simulink model "tut1_screwabouts"  (R2023b)
settings: Solver=VariableStepAuto  StartTime=0.0  StopTime=60  RelTol=1e-3
model workspace (MAT data in the model file):
  c = 1
  m = 1000
libraries: slpidlib x1, simulink x1
settings Model: Creator=Matthew  LastModifiedBy=Matthew

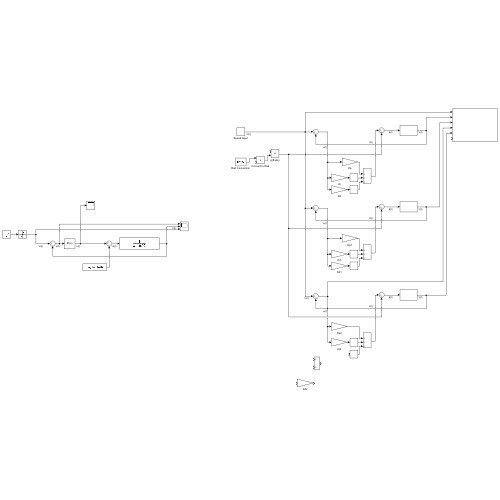
[thumbnail: Simulink's stored preview of the top-level diagram]
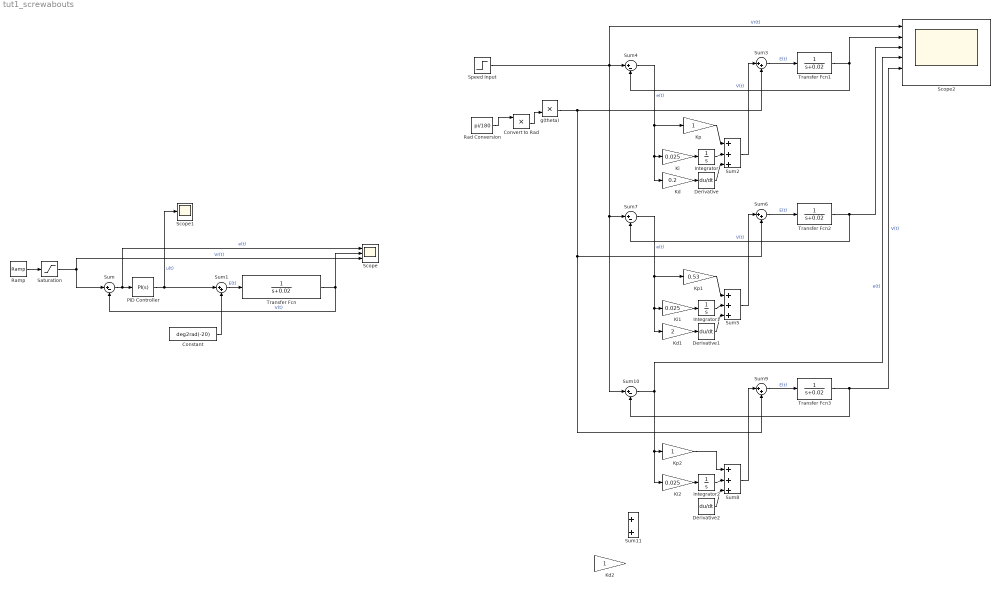
== system tut1_screwabouts ==
  Constant : Constant  Value=deg2rad(-20)
  Convert to Rad : Product
  Derivative : Derivative
  Derivative1 : Derivative
  Derivative2 : Derivative
  Integrator : Integrator
  Integrator1 : Integrator
  Integrator2 : Integrator
  Kd : Gain  Gain=0.2
  Kd1 : Gain  Gain=2
  Kd2 : Gain
  Ki : Gain  Gain=0.025
  Ki1 : Gain  Gain=0.025
  Ki2 : Gain  Gain=0.025
  Kp : Gain
  Kp1 : Gain  Gain=0.53
  Kp2 : Gain
  PID Controller : slpidlib/PID Controller  Controller=PI  Form=Parallel  TimeDomain=Continuous-time  UseExternalTs=off  SampleTime=-1  IntegratorMethod=Forward Euler  FilterMethod=Forward Euler  ControllerParametersSource=internal  P=1.81  I=1.47  UseKiTs=off  D=0  N=0  UseFilter=on  TunerSelectOption=Transfer Function Based (PID Tuner App)  InitialConditionSource=internal  InitialConditionForIntegrator=0  InitialConditionForFilter=0  DifferentiatorICPrevScaledInput=0  ExternalReset=none  TrackingMode=off  Kt=1  LimitOutput=off  SatLimitsSource=internal  UpperSaturationLimit=10  LowerSaturationLimit=-10  LinearizeAsGain=on  AntiWindupMode=none  Kb=1  LimitIntegrator=off  UpperIntegratorSaturationLimit=inf  LowerIntegratorSaturationLimit=-inf  POutMin=[]  POutMax=[]  IOutMin=[]  IOutMax=[]  DOutMin=[]  DOutMax=[]  NOutMin=[]  NOutMax=[]  SumOutMin=[]  SumOutMax=[]  SaturationOutMin=[]  SaturationOutMax=[]  PParamMin=[]  PParamMax=[]  IParamMin=[]  IParamMax=[]  DParamMin=[]  DParamMax=[]  NParamMin=[]  NParamMax=[]  KbParamMin=[]  KbParamMax=[]  KtParamMin=[]  KtParamMax=[]  KbOutMin=[]  KbOutMax=[]  KtOutMin=[]  KtOutMax=[]  IntegratorOutMin=[]  IntegratorOutMax=[]  FilterOutMin=[]  FilterOutMax=[]  SumI1OutMin=[]  SumI1OutMax=[]  SumI2OutMin=[]  SumI2OutMax=[]  SumI3OutMin=[]  SumI3OutMax=[]  SumI4OutMin=[]  SumI4OutMax=[]  SumDOutMin=[]  SumDOutMax=[]  DifferentiatorOutMin=[]  DifferentiatorOutMax=[]  FilterDiffOutCoefMin=[]  FilterDiffOutCoefMax=[]  ReciprocalOutMin=[]  ReciprocalOutMax=[]  SumDenOutMin=[]  SumDenOutMax=[]  SumNumOutMin=[]  SumNumOutMax=[]  DivideOutMin=[]  DivideOutMax=[]  UdiffTsProdOutMin=[]  UdiffTsProdOutMax=[]  NTsProdOutMin=[]  NTsProdOutMax=[]  UintegralTsProdOutMin=[]  UintegralTsProdOutMax=[]  UngainTsProdOutMin=[]  UngainTsProdOutMax=[]  ClampingZeroOutDataTypeStr=Inherit: Inherit via back propagation  ClampingZeroOutMin=[]  ClampingZeroOutMax=[]  FilterDenConstantOutDataTypeStr=Inherit: Inherit via back propagation  FilterDenConstantOutMin=[]  FilterDenConstantOutMax=[]  PCopyOutDataTypeStr=Inherit: Inherit via back propagation  PCopyOutMin=[]  PCopyOutMax=[]  NCopyOutDataTypeStr=Inherit: Inherit via back propagation  NCopyOutMin=[]  NCopyOutMax=[]  IntegratorContinuousStateAttributes=''  IntegratorStateMustResolveToSignalObject=off  IntegratorRTWStateStorageClass=Auto  FilterContinuousStateAttributes=''  FilterStateMustResolveToSignalObject=off  FilterRTWStateStorageClass=Auto  ParallelPVariant=InternalParameters  IdealPVariant=Disabled  IVariant=InternalParameters  DVariant=Disabled  IntegratorVariant=Continuous  SatVariant=Disabled  AWVariant=Passthrough  PCopyVariant=Disabled  TRVariant=Disabled  FdbkBlocksVariant=Forward  IdealPFdbkVariant=Disabled  SatFdbkVariant=Disabled  DerivativeFilterVariant=Disabled  NVariant=Disabled  NCopyVariant=Disabled_SignalSpec  FilterICVariant=Disabled  IntegratorICVariant=InternalICs  ExternalResetVariant=Disabled  TRSumVariant=Passthrough  SumFdbkVariant=Disabled  SumVariant=Sum_PI  TsampFilterVariant=InternalTs  TsampNgainVariant=Passthrough  TsampIntegralVariant=Disabled_SignalSpec  ExternalSaturationOutDataTypeStr=Inherit: Same as second input
  Rad Conversion : Constant  Value=pi/180
  Ramp : simulink/Sources/Ramp  slope=6.8966  start=0  InitialOutput=0  VectorParams1D=off
  Saturation : Saturate  UpperLimit=30  LowerLimit=0
  Scope : Scope  NumInputPorts=3
  Scope1 : Scope
  Scope2 : Scope  NumInputPorts=6
  Speed Input : Step  Time=10  Before=10  After=30  SampleTime=0.1
  Sum{,4,7,10} (4 alike) : Sum  Inputs=|+-
  Sum{1,3,6,9} (4 alike) : Sum  Inputs=|++
  Sum11 : Sum  Inputs=+|+
  Sum2 : Sum  Inputs=|+++
  Sum5 : Sum  Inputs=|+++
  Sum8 : Sum  Inputs=|+++
  Transfer Fcn{,1..3} (4 alike) : TransferFcn  Denominator=[1 0.02]
  g(theta) : Product
  wires:
  Saturation/1 -> Sum/1, Scope/3  "Vr(t)"
  Sum/1 -> Scope/1, PID Controller/1  "e(t)"
  PID Controller/1 -> Sum1/1, Scope1/1  "u(t)"
  Constant/1 -> Sum1/2
  Sum1/1 -> Transfer Fcn/1  "E(t)"
  Transfer Fcn/1 -> Sum/2, Scope/2  "V(t)"
  Ki/1 -> Integrator/1
  Kd/1 -> Derivative/1
  Kp/1 -> Sum2/1
  Integrator/1 -> Sum2/2
  Derivative/1 -> Sum2/3
  Sum4/1 -> Kd/1, Ki/1, Kp/1  "e(t)"
  Sum3/1 -> Transfer Fcn1/1  "E(t)"
  Convert to Rad/1 -> g(theta)/2
  Rad Conversion/1 -> Convert to Rad/1
  Transfer Fcn1/1 -> Sum4/2, Scope2/2  "V(t)"
  Sum2/1 -> Sum3/1
  Sum5/1 -> Sum6/1
  Sum7/1 -> Kd1/1, Ki1/1, Kp1/1  "e(t)"
  Transfer Fcn2/1 -> Scope2/3, Sum7/2  "V(t)"
  Sum6/1 -> Transfer Fcn2/1  "E(t)"
  Ki1/1 -> Integrator1/1
  Kp1/1 -> Sum5/1
  Integrator1/1 -> Sum5/2
  Derivative1/1 -> Sum5/3
  Kd1/1 -> Derivative1/1
  g(theta)/1 -> Sum3/2, Sum9/2, Sum6/2
  Speed Input/1 -> Sum4/1, Scope2/1, Sum10/1, Sum7/1  "Vr(t)"
  Integrator2/1 -> Sum8/2
  Ki2/1 -> Integrator2/1
  Transfer Fcn3/1 -> Scope2/5, Sum10/2  "V(t)"
  Derivative2/1 -> Sum8/3
  Sum8/1 -> Sum9/1
  Sum10/1 -> Scope2/4, Ki2/1, Kp2/1  "e(t)"
  Sum9/1 -> Transfer Fcn3/1  "E(t)"
  Kp2/1 -> Sum8/1
  Ramp/1 -> Saturation/1
